simulink model "HEV_Model_PCT"  (R2014a)
settings: Solver=ode15s  StartTime=0.0  StopTime=195  RelTol=1e-5  AbsTol=1e-4
PreLoadFcn:
  | load UrbanCycle1
  | load UrbanCycle2
  | load UrbanCycle3
  | load UrbanCycle4
  | load UrbanCycle5
  | 
  | assignin('base','decimation',1)
  | Pbatt = 21e3;
  | Vbatt =100;
  | Ts = 6e-5;   % time step
  | 
  | Drive_Cycle_Num = 1;
PostLoadFcn:
  | warning off Simulink:SL_UsingDefaultMaxStepSize
  | warning off Simulink:blocks:MatchingGotoNotFound
  | warning off Simulink:blocks:MatchingFromNotFound
  | warning off Simulink:blocks:TDelayBufferTooSmall
  | warning off Simulink:SL_SaveWithParameterizedLinks_Warning
  | warning off Simulink:SL_TDelayBufferTooSmall
  | warning off ne_sli:nesl_compile:SolverNotRecommended
  | warning off Simulink:SL_OutputNotConnected
  | warning off Simulink:SL_SetParamLinkChangeWarn
  | warning off Simulink:SL_SaveWithDisabledLinks_Warning
  | warning('off','Simulink:SL_UINotUpdatedDuringRapidAccelSim');
  | warning off Simulink:Engine:OutputNotConnected
  | warning off Simulink:Engine:UINotUpdatedDuringRapidAccelSim
  | warning off Simulink:Engine:SaveWithParameterizedLinks_Warning
  | warning off Simulink:Engine:SolverMaskedZC
  | set_param(bdroot,'MaskedZcDiagnostic','none');
  | warning off Simulink:Engine:SolverInconsistentInitialConditionsWarnForDAE
  | set_param(bdroot,'IgnoredZcDiagnostic','none');
  | warning off Simulink:Engine:SolverIgnoredZCBracketing
  | set_param(bdroot,'MaxConsecutiveZCsMsg','none');
  | warning off Simulink:Engine:SolverConsecutiveZCNum
  | warning off Simulink:Engine:SolverMinStepSizeWarnForDAE
  | 
  | %Setup_HEV_Model_Configurations
InitFcn:
  | %Configure_HEV_Simulation
model workspace (MAT data in the model file):
  guiH = 18054.0001221
undefined symbols (not defined in the file or in its folder): drive_block, drive_enginemodel, HEV_Param, HEV_Vehicle_Dynamics_Lib, sigbuilder_block, Simple, speed, torque
undefined symbols (not defined in the file): HEV_Vehicle_Mass
libraries: fl_lib x34, nesl_utility x16, sdl_lib x2, simulink x1, HEV_Electrical_Lib x1, TunableMech_lib x1, powerlib x1
(part 1 of 2)
Description:
  | Copyright 2008 The MathWorks(TM), Inc.
settings Model: ExtModeAutoUpdateStatusClock=off  TunableVars=Drive_Cycle_Num,HEV_Vehicle_Mass  TunableVarsStorageClass=Auto,Auto  TunableVarsTypeQualifier=,  BufferReuse=off  Creator=tegel  LastModifiedBy=smiller
settings SolverCC: ZcThreshold=0  ZeroCrossAlgorithm=Adaptive
settings DataIOCC: SignalLoggingSaveFormat=ModelDataLogs  DSMLogging=off
settings OptimizationCC: InlineParams=on  OptimizeBlockIOStorage=off  BufferReuse=off  GlobalBufferReuse=off  ExpressionFolding=off  ExpressionDepthLimit=2147483647  LocalBlockOutputs=off  InitFltsAndDblsToZero=on  EfficientMapNaN2IntZero=off
settings DebuggingCC: AlgebraicLoopMsg=error  UnderspecifiedInitializationDetection=Classic  SignalResolutionControl=TryResolveAllWithWarning  MaxConsecutiveZCsMsg=none  MaskedZcDiagnostic=none  IgnoredZcDiagnostic=none  MultiTaskDSMMsg=warning  MultiTaskCondExecSysMsg=none  SigSpecEnsureSampleTimeMsg=none  FcnCallInpInsideContextMsg=UseLocalSettings  UnknownTsInhSupMsg=none  StateNameClashWarn=warning
settings HardwareCC: TargetLongLongMode=on  TargetEndianess=LittleEndian  TargetHWDeviceType=MATLAB Host  ProdEqTarget=off
settings SFSimCC: SimParseCustomCode=off
settings GRTTargetCC: CombineOutputUpdateFcns=off  GRTInterface=on

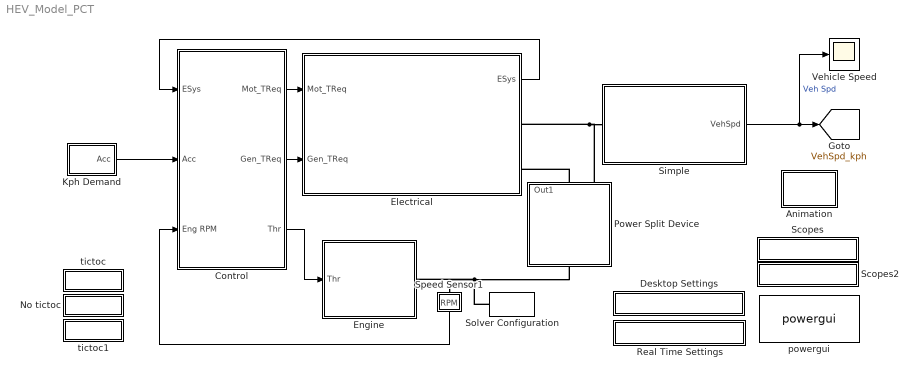
== system HEV_Model_PCT ==
  Animation : Subsystem  BlockChoice=Off
      mask init:
      | Configure_HEV_Animation
      settings: AttributesFormatString=%<BlockChoice>  TemplateBlock=Animation_Lib/Animation  MemberBlocks=Off,On
  Control : Subsystem
      mask Display:
      | image(imread('HEV_Control_IMAGE.jpg'));
      | port_label('input',1,'ESys');
      | port_label('input',2,'Acc');
      | port_label('input',3,'Eng RPM');
      | port_label('output',1,'Mot_TReq');
      | port_label('output',2,'Gen_TReq');
      | port_label('output',3,'Thr');
  Desktop Settings : Subsystem
      settings: OpenFcn=|
      | set_param(bdroot,'Solver','ODE15s');
      | 
      | %set_param([bdroot '/Electrical'],'MaskInitialization','Configure_HEV_Simulation');
      | 
      | %set_param([bdroot '/Animation'],'MaskInitialization','Configure_HEV_Simulation');
      | 
      | HEV_Param.Control.Mode_Logic_TS = 0.1;
      | 
      | tvar_solverBlock = find_system(bdroot,'FollowLinks','on','LookUnderMasks','on', 'SubClassName', 'solver');
      | 
      | for i=1:size(tvar_solverBlock,1)
      | 
      | set_param(char(tvar_solverBlock(i)), 'UseLocalSolver','off','DoFixedCost','off');
      | end
      | 
      | clear tvar_solverBlock
      mask Display: disp('Desktop Settings')
  Electrical : Subsystem  BlockChoice=System Level
      link override Detailed/Battery: BlockChoice=Predefined
      link override System Level/Battery: BlockChoice=Generic
      link override System Level/Battery/Predefined/Intf: T=100000
      link override System Level/Battery/Predefined/Preset Battery: SOC=HEV_Param.Battery_Det.Initial_SOC  MaxQ=8.1  FullV=232.7974  Dis_rate=3.5217  R=0.24691  Normal_OP=7.3252  expZone="[216.0772     0.3979565]"  Dis_Char=off  NomV=HEV_Param.Battery_Det.Nominal_Voltage  BatType=Nickel-Metal-Hydride
      mask init:
      | %disp('Elec Mask Init');
      | Configure_HEV_Simulation
      settings: AttributesFormatString=%<BlockChoice>  TemplateBlock=HEV_Electrical_Lib/Electrical  MemberBlocks=Detailed,Mean Value,System Level
  Engine : Subsystem
      mask Display:
      | image(imread('HEV_Engine_IMAGE.jpg'));
      | port_label('input',1,'Thr');
      | port_label('RConn',1,'Sh');
  Kph Demand : Subsystem
      mask Display:
      | plotstr=['UrbanCycle' evalin('base','num2str(Drive_Cycle_Num)')];
      | plot(evalin('base',[plotstr '.time']),evalin('base',[plotstr '.SpdKph']));
      | text(evalin('base',['0.7*max(' plotstr '.time)']),evalin('base',['0.25*max(' plotstr '.SpdKph)']),evalin('base','num2str(Drive_Cycle_Num)'));
  No tictoc : Subsystem
      settings: OpenFcn=|
      | set_param(bdroot,'StartFcn','');
      | set_param(bdroot,'StopFcn','');
      mask Display: disp('No tictoc')
  "Power Split Device " : Subsystem
      mask Display:
      | image(imread('HEV_Planetary_Gear_IMAGE.jpg'));
      | color('black');
      | port_label('Lconn',1,'C');
      | port_label('Rconn',1,'S');
      | port_label('Rconn',2,'R');
  Real Time Settings : Subsystem
      settings: OpenFcn=|
      | tvar_Nonlinear_Iterations = '3';
      | tvar_StepSize = '0.005';                                                                                                                                                                               Select_HEV_Model_Systems('Sys BC VS',HEV_Configs);
      | 
      | %tvar_LocalSolver = 'NE_TRAPEZOIDAL_ADVANCER';
      | tvar_LocalSolver = 'NE_BACKWARD_EULER_ADVANCER';
      | 
      | set_param([bdroot '/Electrical'],'MaskInitialization','%Configure_HEV_Simulation');                                                                                                                set_param([bdroot '/Animation'],'MaskInitialization','%Configure_HEV_Simulation');
      | 
      | HEV_Param.Control.Mode_Logic_TS = str2num(tvar_StepSize);
      | 
      | set_param(bdroot,'Solver','ode1','FixedStep','auto');
      | tvar_solverBlock = find_system(bdroot,'FollowLinks','on','LookUnderMasks','on', 'SubClassName', 'solver');
      | for i=1:size(tvar_solverBlock,1)
      | 
      | 
      |     set_param(char(tvar_solverBlock(i)), 'UseLocalSolver','on','DoFixedCost','on','MaxNonlinIter',tvar_Nonlinear_Iterations,'LocalSolverChoice',tvar_LocalSolver,'LocalSolverSampleTime',tvar_StepSize);
      | end
      | clear tvar_Nonlinear_Iterations tvar_StepSize tvar_LocalSolver tvar_solverBlock
      mask Display: disp('Real Time Settings')
  Scopes : Subsystem  mask(Data Acquisition){}
      mask Display: disp('Scopes');
  Scopes2 : Subsystem  mask(Data Acquisition){}
      mask Display: disp('Fuel Economy');
  Simple : Subsystem  AncestorBlock=HEV_Vehicle_Dynamics_Lib/Simple  mask(Rigid vehicle model){mass=HEV_Vehicle_Mass, area=HEV_Param.Vehicle.Frontal_Area, Cd=HEV_Param.Vehicle.Aero_Drag_Coeff, radius=HEV_Param.Vehicle.Tire_Radius, wheel_inertia=HEV_Param.Vehicle.Wheel_Inertia, gear_ratio=HEV_Param.Vehicle.Engine_Vehicle_Gear_Ratio}
      mask prompts: mass "Vehicle mass (Kg)"; area "Vehicle Area (m^2)"; Cd "Aerodynamic drag coefficient (unitless)"; radius "Tire radius (m)"; wheel_inertia "Total wheel inertia (kg*m^2)"; gear_ratio "Engine to vehicle gear ratio"
      mask help:
      | Model vehicle effective inertia and drag force as seen by the engine. It
      | is assumed that the vehicle is moving on flat terrain. No bearing friction
      | or gear losses are included.
      mask init:
      | gravity = 9.81;
      mask Display:
      | image(imread('HEV_Vehicle_Dynamics_Simple_IMAGE.jpg'));
      | port_label('LConn',1,'Sh');
      | port_label('output',1,'Spd');
  Solver Configuration : nesl_utility/Solver Configuration  PhysicalDomain=network_engine_domain  SubClassName=solver  LeftPortType=input  RightPortType=generic  Accelerate=off  Tones=[]  Harmonics=[]  SimulateNoise=off  Profile=off  UseLocalSampling=off  EnableSwitchedLinearOptims=on  FrequencyDomain=off  UseCCode=off  RelTol=0.001  AbsTol=1e-06  MinStep=1e-09  ToWorkspace=off  DoDC=off  ResidualTolerance=1e-8  UseLocalSolver=off  LocalSolverChoice=NE_BACKWARD_EULER_ADVANCER  LocalSolverSampleTime=0.005  DoFixedCost=off  MaxNonlinIter=3  MaxModeIter=2  LinearAlgebra=Sparse  DelaysMemoryBudget=1024  AutomaticFiltering=on  FilteringTimeConstant=0.001
  Speed Sensor1 : Subsystem
      mask Display: disp('S')
  Vehicle Speed : Scope
      settings: YMin=-20  YMax=120  Decimation=decimation
  powergui : powerlib/powergui  SimulationMode=Continuous  SolverType=Tustin  SampleTime=Ts  frequency=60  SPID=on  DisableSnubberDevices=off  DisableRonSwitches=off  DisableVfSwitches=off  SwTol=0  Interpol=off  DisplayEquations=off  Ts=0  methode=off  frequencyindice=0  Pbase=100e6  ErrMax=1e-4  Iterations=50  UnitsV=kV  UnitsW=MW  FunctionMessages=off  echomessages=off  HookPort=off  EnableUseOfTLC=off  x0status=blocks  RestoreLinks=warning  ResistiveCurrentMeasurement=off  Frange=[0:2:500]  Ylog=off  Xlog=on  ShowGrid=off  save=off  variable=ZData  structure=0  ZoomFFT=on  StartTime=0.0  cycles=1  DisplayStyle=1  fundamental=60  FreqAxis=off  MaxFrequency=1000  frequencyindicesteady=1  RmsSteady=1  display=off
  tictoc : Subsystem
      settings: OpenFcn=|
      | set_param(bdroot,'StartFcn','tic;');
      | set_param(bdroot,'StopFcn','Elapsed_Sim_Time = toc; disp([''Elapsed time is '' num2str(Elapsed_Sim_Time)])');
      mask Display: disp('tictoc')
  tictoc1 : Subsystem
      settings: OpenFcn=open('HEV_Model_Demo_Script.html')
      mask Display: disp('Script')
  tag scope: VehSpd_kph=global
  wires:
  Simple/1(VehSpd) -> [VehSpd_kph], Vehicle Speed/1  "Veh Spd"
  Speed Sensor1/1(RPM) -> Control/3(Eng RPM)
  Control/1(Mot_TReq) -> Electrical/1(Mot_TReq)
  Control/2(Gen_TReq) -> Electrical/2(Gen_TReq)
  Control/3(Thr) -> Engine/1(Thr)
  Kph Demand/1(Acc) -> Control/2(Acc)
  Electrical/1(ESys) -> Control/1("ESys ")
  connections:
  "Power Split Device "/RConn1 -- Electrical/RConn2
  Simple/LConn1 -- "Power Split Device "/RConn2 -- Electrical/RConn1
  Engine/RConn1 -- Speed Sensor1/LConn1 -- "Power Split Device "/LConn1 -- Solver Configuration/RConn1

== system HEV_Model_PCT/Animation ==
  Off : Subsystem

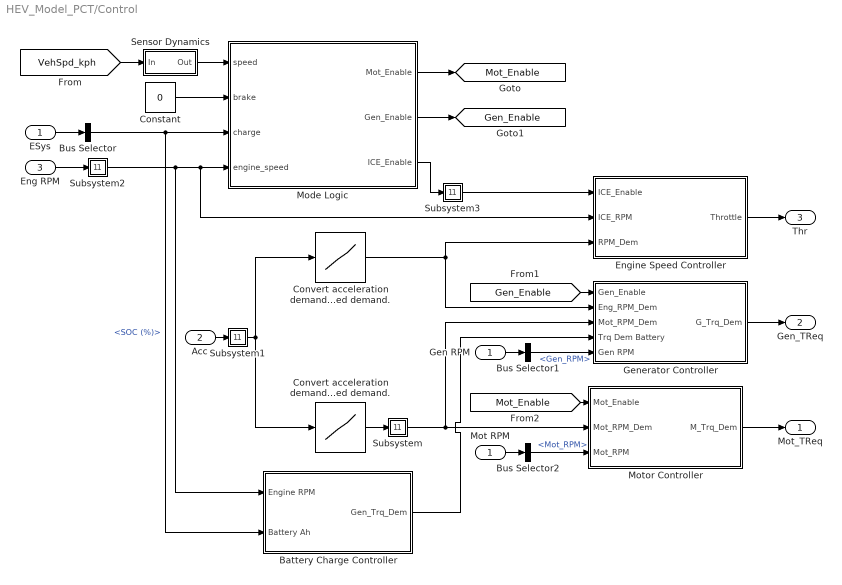
== system HEV_Model_PCT/Control ==
  "ESys " : Inport
  Acc : Inport  Port=2
  Eng RPM : Inport  Port=3
  Battery Charge Controller : Subsystem
  Bus Selector : BusSelector  OutputSignals=Batt.SOC (%)
  Bus Selector1 : BusSelector  OutputSignals=Gen_RPM
  Bus Selector2 : BusSelector  OutputSignals=Mot_RPM
  Constant : Constant  Value=0
  Convert acceleration demand to engine speed demand. : Lookup  InputValues=[0 0.1 1]  Table=[0 800 4000]
  Convert acceleration demand to motor speed demand. : Lookup  InputValues=[0 1]  Table=[0 2500]
  Engine Speed Controller : Subsystem
  Gen RPM : InportShadow
  Generator Controller : Subsystem
  Mode Logic : Stateflow chart  TreatAsAtomicUnit=on
  Mot RPM : InportShadow
  Motor Controller : Subsystem
  Sensor Dynamics : Subsystem  mask(First-order lag supporting vector signals){b=HEV_Param.ICE.sensor_time_constant, x_initial=0}
      mask prompts: b "Filter time constant"; x_initial "Initial output"
      mask help: Models a lag of the form 1/(b*s+1) where s is the Laplace operator.
  Subsystem : Subsystem
      mask Display: disp('S')
  Subsystem1 : Subsystem
      mask Display: disp('S')
  Subsystem2 : Subsystem
      mask Display: disp('S')
  Subsystem3 : Subsystem
      mask Display: disp('S')
  Mot_TReq : Outport
  Gen_TReq : Outport  Port=2
  Thr : Outport  Port=3
  tag scope: Gen_Enable=global, Mot_Enable=global
  wires:
  Acc/1 -> Subsystem1/1(In1)
  Eng RPM/1 -> Subsystem2/1(In1)
  Engine Speed Controller/1(Throttle) -> Thr/1
  Convert acceleration demand to motor speed demand./1 -> Subsystem/1(In1)
  Convert acceleration demand to engine speed demand./1 -> Engine Speed Controller/3(RPM_Dem), Generator Controller/2(Eng_RPM_Dem)
  Bus Selector2/1 -> Motor Controller/3(Mot_RPM)  "<Mot_RPM>"
  Motor Controller/1(M_Trq_Dem) -> Mot_TReq/1
  Generator Controller/1(G_Trq_Dem) -> Gen_TReq/1
  "ESys "/1 -> Bus Selector/1
  Subsystem2/1(Eng_RPM_Meas) -> Battery Charge Controller/1(Engine RPM), Mode Logic/4(engine_speed), Engine Speed Controller/2(ICE_RPM)
  Bus Selector/1 -> Battery Charge Controller/2(Battery Ah), Mode Logic/3(charge)  "<SOC (%)>"
  Constant/1 -> Mode Logic/2(brake)
  Mode Logic/3(ICE_Enable) -> Subsystem3/1(In1)
  Subsystem3/1(Gen_RPM_Dem) -> Engine Speed Controller/1(ICE_Enable)
  Mode Logic/2(Gen_Enable) -> [Gen_Enable]
  Mode Logic/1(Mot_Enable) -> [Mot_Enable]
  Sensor Dynamics/1(Out) -> Mode Logic/1(speed)
  Bus Selector1/1 -> Generator Controller/5(Gen RPM)  "<Gen_RPM>"
  Subsystem/1(Motor_RPM_Dem) -> Motor Controller/2(Mot_RPM_Dem), Generator Controller/3(Mot_RPM_Dem)
  [Gen_Enable] -> Generator Controller/1(Gen_Enable)
  [Mot_Enable] -> Motor Controller/1(Mot_Enable)
  Battery Charge Controller/1(Gen_Trq_Dem) -> Generator Controller/4(Trq Dem Battery)
  Gen RPM/1 -> Bus Selector1/1
  Mot RPM/1 -> Bus Selector2/1
  Subsystem1/1(Accel) -> Convert acceleration demand to motor speed demand./1, Convert acceleration demand to engine speed demand./1
  [VehSpd_kph] -> Sensor Dynamics/1(In)

== system HEV_Model_PCT/Desktop Settings ==

== system HEV_Model_PCT/Electrical ==
  Mot_TReq : Inport
  Gen_TReq : Inport  Port=2
  System Level : HEV_Electrical_Lib/System Level  SystemSampleTime=-1
  Mot_Sh : PMIOPort  Port=1  Side=Right
  Gen_Sh : PMIOPort  Port=2  Side=Right
  ESys : Outport
  wires:
  Mot_TReq/1 -> System Level/1
  Gen_TReq/1 -> System Level/2
  System Level/1 -> ESys/1
  connections:
  System Level/RConn1 -- Mot_Sh/RConn1
  System Level/RConn2 -- Gen_Sh/RConn1

== system HEV_Model_PCT/Engine ==
  Thr : Inport
  Generic Engine : sdl_lib/Engines/Generic Engine  model_parameterization=1  engine_type=1  P_max=HEV_Param.ICE.Max_Power W  w_P_max=HEV_Param.ICE.Speed_At_Max_Power rpm  w_max=HEV_Param.ICE.Max_Speed rpm  w_min=500 rpm  w_tab=[ 500 1000 2e+3 3e+3 4e+3 5e+3 6e+3 7e+3 ] rpm  trq_tab=[ 380 380 380 380 350 280 200 80 ] N*m  pwr_tab=[ 2e+4 4e+4 7.8e+4 1.2e+5 1.45e+5 1.48e+5 1.25e+5 6e+4 ] W  interp_method=1  model_inertia=0  inertia=1 kg*m^2  initial_velocity=800 rpm  model_time_constant=0  time_constant=0.2 s  T0=0  w_thr=100 rpm  idle_speed=0  idle_speed_reference=1000 rpm  tau_controller=1 s  idle_w_thr=1 rpm  fc_model=1  fc_per_rev=25 mg/rev  displaced_volume=400 cm^3  rev_per_cycle=2  fc_w_tab=[ 1000 2e+3 3e+3 4e+3 5e+3 6e+3 ] rpm  fc_trq_tab=[ 0 80 160 200 240 320 360 400 ] N*m  fc_tab=[ 0.5 0.9 1.4 1.6 1.9 2.7 3.4 4.4; 1 1.7 2.7 3.1 3.6 5 6 7.4; 1.4 2.7 4 4.8 5.6 7.5 8.5 10.5; 2 3.6 5.8 6.7 8 10.4 11.7 13.3; 2.5 4.8 7.9 9.4 10.8 14 16.2 18.6; 3.1 6 10.3 11.9 13.8 18.4 22 26.5 ] g/s  bmep_tab=[ 0 250 500 625 750 1000 1.15e+3 1.25e+3 ] kPa  bsfc_tab=[ 410 380 300 280 270 290 320 380; 410 370 290 270 260 270 285 320; 415 380 290 275 265 270 270 300; 420 390 310 290 285 280 280 285; 430 410 340 320 310 300 310 320; 450 430 370 340 330 330 350 380 ] g/hr/kW  fc_interp_method=1
  Inertia1 : fl_lib/Mechanical/Rotational Elements/Inertia  inertia=HEV_Param.ICE.Shaft_Inertia kg*m^2  w_specify=on  w_priority=High  w=0 rad/s  t_specify=off  t_priority=High  t=0 N*m
  Mechanical Rotational Reference : fl_lib/Mechanical/Rotational Elements/Mechanical Rotational Reference
  Mechanical Rotational Reference1 : fl_lib/Mechanical/Rotational Elements/Mechanical Rotational Reference
  Rotational Damper : fl_lib/Mechanical/Rotational Elements/Rotational Damper  D=HEV_Param.ICE.Friction N*m/(rad/s)  w_specify=off  w_priority=High  w=0 rad/s  t_specify=off  t_priority=High  t=0 N*m
  Sensor : Subsystem
      mask Display: disp('S');
  Simulink-PS Converter : nesl_utility/Simulink-PS Converter  PhysicalDomain=network_engine_domain  SubClassName=ps_input  LeftPortType=input  RightPortType=output  PseudoPeriodic=off  Frequencies=[]  NoiseDistribution=none  NoiseParameters=[]  Unit=1  AffineConversion=off  InputFiltering=off  SimscapeFilterOrder=1  InputFilterTimeConstant=.001  UdotUserProvided=0
  Sh : PMIOPort  Port=1  Side=Right
  wires:
  Thr/1 -> Simulink-PS Converter/1  "Throttle"
  connections:
  Sensor/RConn1 -- Sh/RConn1
  Mechanical Rotational Reference1/LConn1 -- Rotational Damper/RConn1
  Simulink-PS Converter/RConn1 -- Generic Engine/LConn1
  Mechanical Rotational Reference/LConn1 -- Generic Engine/LConn2
  Sensor/LConn1 -- Generic Engine/RConn3 -- Inertia1/LConn1 -- Rotational Damper/LConn1

== system HEV_Model_PCT/Kph Demand ==
  "10-15 mode " : Subsystem  Tag=STV Subsys  LoadFcn=sigbuilder_block('load');  StartFcn=sigbuilder_block('start');  StopFcn=sigbuilder_block('stop');  ClipboardFcn=sigbuilder_block('clipboard');  mask(Sigbuilder block){}
      mask help: Sigbuilder GUI
      mask init:
      | if ~strcmp(get_param(bdroot(gcbh),'SimulationStatus'),'stopped') tuvar = sigbuilder_block('maskInit'); end
      settings: CopyFcn=sigbuilder_block('copy');  DeleteFcn=sigbuilder_block('delete');  ModelCloseFcn=sigbuilder_block('modelClose');  PreSaveFcn=sigbuilder_block('preSave');  PauseFcn=sigbuilder_block('pause')  ContinueFcn=sigbuilder_block('continue')  NameChangeFcn=sigbuilder_block('namechange');  OpenFcn=sigbuilder_block('open',[561.75 178.5 550.5 399 ]);  CloseFcn=sigbuilder_block('close');
      mask Display: plot(0,0,100,100,[10,10,40,40,10],[80,20,20,80,80],[40,10],[50,50], [40,27,10],[65,72,56],[40,25,25,10],[28,28,43,43]);
  FTP75 : FromWorkspace  VariableName=[UrbanCycle4.time UrbanCycle4.SpdKph]  SampleTime=0
  Multiport Switch : MultiPortSwitch  Inputs=5
  Select Cycle : Constant  Value=Drive_Cycle_Num
  Urban Cycle 1 : FromWorkspace  VariableName=[UrbanCycle1.time UrbanCycle1.SpdKph]  SampleTime=0
  Urban Cycle 2 : FromWorkspace  VariableName=[UrbanCycle2.time UrbanCycle2.SpdKph]  SampleTime=0
  Urban Cycle 3 : FromWorkspace  VariableName=[UrbanCycle3.time UrbanCycle3.SpdKph]  SampleTime=0
  Vehicle Speed Controller : Subsystem
  Acc : Outport
  wires:
  Urban Cycle 3/1 -> Multiport Switch/4
  Select Cycle/1 -> Multiport Switch/1
  Urban Cycle 2/1 -> Multiport Switch/3
  Urban Cycle 1/1 -> Multiport Switch/2
  Vehicle Speed Controller/1(Acc) -> Acc/1
  Multiport Switch/1 -> Vehicle Speed Controller/1(Ref Spd)
  [VehSpd_kph] -> Vehicle Speed Controller/2(Veh Spd)
  FTP75/1 -> Multiport Switch/5
  "10-15 mode "/1(Target speed) -> Multiport Switch/6

== system HEV_Model_PCT/No tictoc ==

== system HEV_Model_PCT/Power Split Device  ==
  note: For port placement
  Constant : Constant
  Planetary Gear : sdl_lib/Gears/Planetary Gear  rs_ratio=HEV_Param.Power_Split.Ratio_Ring2Sun  friction_model=2  efficiency=[ 0.96 0.98 ]  mu_visc=[ 0.02 0 ] N*m/(rad/s)  w_thr=[ 0.01 0.01] rad/s
  Sensor1 : Subsystem
      mask Display: disp('S')
  Sensor2 : Subsystem
      mask Display: disp('S')
  Sensor3 : Subsystem
      mask Display: disp('S')
  S : PMIOPort  Port=1  Side=Right
  R : PMIOPort  Port=2  Side=Right
  C : PMIOPort  Port=3  Side=Left
  Out1 : Outport
  wires:
  Constant/1 -> Out1/1
  connections:
  S/RConn1 -- Sensor3/RConn1
  Planetary Gear/RConn1 -- Sensor2/LConn1
  Planetary Gear/RConn2 -- Sensor3/LConn1
  R/RConn1 -- Sensor2/RConn1
  Sensor1/LConn1 -- C/RConn1
  Sensor1/RConn1 -- Planetary Gear/LConn1

== system HEV_Model_PCT/Real Time Settings ==

== system HEV_Model_PCT/Scopes ==
  Batt Cell Temp : Scope
      settings: YMin=20  YMax=60  SaveName=DCDC_Temp1  MaxDataPoints=100  Decimation=decimation
  Batt DCDC Scopes : Subsystem
  Car Scopes : Subsystem
  DC DC Temp : Scope
      settings: YMin=20  YMax=60  SaveName=DCDC_Temp  MaxDataPoints=100  Decimation=decimation*100
  Demux1 : Demux  Outputs=2
  Drivetrain Scopes : Subsystem
  Electricals Scopes : Subsystem
  ICE Scopes : Subsystem
  Mode Logic : Subsystem
  Motor Generator Scopes : Subsystem
  Speeds (RPM) : Scope  NumInputPorts=2
      settings: YMin=-500~-1000  YMax=1500~5000  SaveName=ScopeData9  MaxDataPoints=100  Decimation=decimation
  Voltages : Scope  NumInputPorts=2
      settings: YMin=490~160  YMax=520~260  MaxDataPoints=100  Decimation=decimation
  wires:
  Electricals Scopes/1(V) -> Demux1/1
  Demux1/1 -> Voltages/1  "DC Bus"
  Demux1/2 -> Voltages/2  "Battery"
  Motor Generator Scopes/1(M) -> Speeds (RPM)/1  "Motor"
  Motor Generator Scopes/2(G) -> Speeds (RPM)/2  "Generator"
  Batt DCDC Scopes/1(DCDC Temp) -> DC DC Temp/1
  Batt DCDC Scopes/2(Batt Cell Temp) -> Batt Cell Temp/1

== system HEV_Model_PCT/Scopes2 ==
  note: Fuel Economy
  (L/100 km) : Display
      settings: Decimation=decimation
  (MPG) : Display
      settings: Decimation=decimation
  (km/L) : Display
      settings: Decimation=decimation
  Calculate Fuel Economy : Subsystem
  Fuel Consumption Table : Lookup2D  RowIndex=HEV_Param.ICE.FC.Speed_Vector  ColumnIndex=HEV_Param.ICE.FC.Torque_Vector  Table=HEV_Param.ICE.FC.Consumption_Table
  Total Fuel Used (L) : Display
      settings: Decimation=decimation
  wires:
  Calculate Fuel Economy/1(Liter/100Km) -> (L/100 km)/1
  Calculate Fuel Economy/3(MPG) -> (MPG)/1
  [VehSpd_kph] -> Calculate Fuel Economy/1(Kph)
  Calculate Fuel Economy/4(Fuel Used (L)) -> Total Fuel Used (L)/1
  Calculate Fuel Economy/2(Km/Liter) -> (km/L)/1
  Fuel Consumption Table/1 -> Calculate Fuel Economy/2(Fuel Flow g/s)
  [EngSpd_RPM] -> Fuel Consumption Table/1
  [Carrier_Trq_Nm] -> Fuel Consumption Table/2

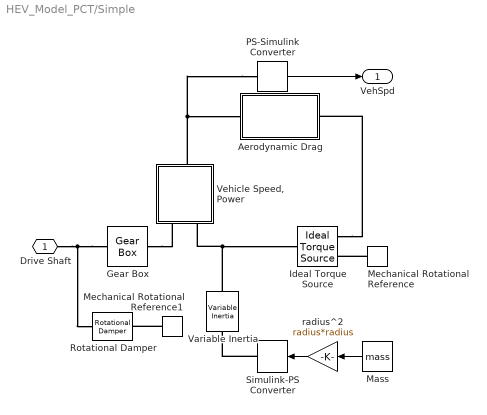
== system HEV_Model_PCT/Simple ==
  Aerodynamic Drag : Subsystem
  Gear Box : fl_lib/Mechanical/Mechanisms/Gear Box  ratio=gear_ratio  t_in_specify=off  t_in_priority=High  t_in=0 N*m  t_out_specify=off  t_out_priority=High  t_out=0 N*m
  Ideal Torque Source : fl_lib/Mechanical/Mechanical Sources/Ideal Torque Source
  Mass : Constant  Value=mass
  Mechanical Rotational Reference : fl_lib/Mechanical/Rotational Elements/Mechanical Rotational Reference
  Mechanical Rotational Reference1 : fl_lib/Mechanical/Rotational Elements/Mechanical Rotational Reference
  PS-Simulink Converter : nesl_utility/PS-Simulink Converter  PhysicalDomain=network_engine_domain  SubClassName=ps_output  LeftPortType=input  RightPortType=output  PseudoPeriodic=off  Frequencies=[]  Unit=1  AffineConversion=off
  Rotational Damper : fl_lib/Mechanical/Rotational Elements/Rotational Damper  D=HEV_Param.Vehicle.Trans.Friction N*m/(rad/s)  w_specify=off  w_priority=High  w=0 rad/s  t_specify=off  t_priority=High  t=0 N*m
  Simulink-PS Converter : nesl_utility/Simulink-PS Converter  PhysicalDomain=network_engine_domain  SubClassName=ps_input  LeftPortType=input  RightPortType=output  PseudoPeriodic=off  Frequencies=[]  NoiseDistribution=none  NoiseParameters=[]  Unit=kg*m*m  AffineConversion=off  InputFiltering=off  SimscapeFilterOrder=1  InputFilterTimeConstant=.001  UdotUserProvided=0
  Variable Inertia : TunableMech_lib/Variable Inertia  initial_velocity=0 rad/s  t_specify=off  t_priority=High  t=0 N*m
  "Vehicle Speed, Power" : Subsystem
  radius^2 : Gain  Gain=radius*radius
  Drive Shaft : PMIOPort  Port=1  Side=Left
  VehSpd : Outport
  wires:
  PS-Simulink Converter/1 -> VehSpd/1
  Mass/1 -> radius^2/1
  radius^2/1 -> Simulink-PS Converter/1
  connections:
  Gear Box/RConn1 -- "Vehicle Speed, Power"/LConn1
  Mechanical Rotational Reference1/LConn1 -- Rotational Damper/RConn1
  Variable Inertia/LConn1 -- "Vehicle Speed, Power"/LConn2 -- Ideal Torque Source/LConn1
  Mechanical Rotational Reference/LConn1 -- Ideal Torque Source/RConn2
  Ideal Torque Source/RConn1 -- Aerodynamic Drag/RConn1
  PS-Simulink Converter/LConn1 -- Aerodynamic Drag/LConn1 -- "Vehicle Speed, Power"/RConn1
  Gear Box/LConn1 -- Drive Shaft/RConn1 -- Rotational Damper/LConn1
  Simulink-PS Converter/RConn1 -- Variable Inertia/RConn1

== system HEV_Model_PCT/Speed Sensor1 ==
  Ideal Rotational Motion Sensor : fl_lib/Mechanical/Mechanical Sensors/Ideal Rotational Motion Sensor  offset=0 rad
  Mechanical Rotational Reference : fl_lib/Mechanical/Rotational Elements/Mechanical Rotational Reference
  PS-Simulink Converter1 : nesl_utility/PS-Simulink Converter  PhysicalDomain=network_engine_domain  SubClassName=ps_output  LeftPortType=input  RightPortType=output  PseudoPeriodic=off  Frequencies=[]  Unit=rpm  AffineConversion=off
  Sensor Dynamics : Subsystem  mask(First-order lag supporting vector signals){b=HEV_Param.ICE.sensor_time_constant, x_initial=0}
      mask prompts: b "Filter time constant"; x_initial "Initial output"
      mask help: Models a lag of the form 1/(b*s+1) where s is the Laplace operator.
  Shaft : PMIOPort  Port=1  Side=Left
  RPM : Outport
  wires:
  PS-Simulink Converter1/1 -> Sensor Dynamics/1(In)
  Sensor Dynamics/1(Out) -> RPM/1
  connections:
  PS-Simulink Converter1/LConn1 -- Ideal Rotational Motion Sensor/RConn2
  Mechanical Rotational Reference/LConn1 -- Ideal Rotational Motion Sensor/RConn1
  Ideal Rotational Motion Sensor/LConn1 -- Shaft/RConn1

== system HEV_Model_PCT/tictoc ==

== system HEV_Model_PCT/tictoc1 ==

== system HEV_Model_PCT/Animation/Off ==

== system HEV_Model_PCT/Control/Battery Charge Controller ==
  Engine RPM : Inport
  Battery Ah : Inport  Port=2
  Allow 20% of available torque to be used to charge the battery : Gain  Gain=-0.2
  Engine Model : Subsystem  DialogController=PMDialogs.PMDefaultMaskDlg  LoadFcn=drive_block('LoadFcn');  StartFcn=drive_enginemodel('Start');  mask(Gasoline Engine){power_max=43e3, speed_at_power_max=4000, speed_max=6000}
      mask prompts: power_max "Maximum power [W]:"; speed_at_power_max "Speed at maximum power [rpm]:"; speed_max "Maximum speed [rpm]:"
      mask help:
      | Simple gasoline fuel engine model with speed governor.  The throttle input signal lies between zero and one and specifies the torque demanded from the engine as a fraction of the maximum possible torque.  This signal also indirectly controls the engine speed.  The engine model does not include air-fuel combustion dynamics.
      |
      | If the throttle signal rises above one or falls below zero, the engine limits the signal to one or zero, respectively. If the engine speed rises above the maximum speed, the engine torque drops to zero.
      mask init:
      | drive_preinitmask();[speed,power,torque,p] = ...
      | 	drive_enginemodel('MaskGasoline');
      settings: CopyFcn=drive_block('CopyFcn');  DeleteFcn=drive_block('DeleteFcn');  PreSaveFcn=drive_block('PreSaveFcn');  PostSaveFcn=drive_block('PostSaveFcn');  PreCopyFcn=drive_block('PreCopyFcn');  PreDeleteFcn=drive_block('PreDeleteFcn');
      mask Help: web(drive_help);
      mask Display:
      | image(imread('engine.bmp'),'center')
      | plot(speed, torque/max(torque))
      | plot(speed, power/max(power))
      | port_label('input', 1, 'RPM')
      | port_label('output', 1, 'Tmax')
  Engine-generator gear ratio : Gain  Gain=1/2
  "If the battery has more than 100% rated capacity, then no generation is required. Linearly ramp to using 20% of engine torque for charging between 50% capacity and 100% capacity." : Lookup  InputValues=[0 50 100 150]  Table=[-5 -5 0 0]
  Max : Constant  Value=5
  Nm2Volts : Gain  Gain=5/400
  Saturation Dynamic : simulink/Discontinuities/Saturation Dynamic  OutMin=[]  OutMax=[]  OutDataTypeStr=Inherit: Same as second input  OutDataType=sfix(16)  OutScaling=2^-10  DoSatur=off
  Volts2Nm : Gain  Gain=400/5
  Gen_Trq_Dem : Outport
  tag scope: gen_torque_dem=global
  wires:
  Battery Ah/1 -> "If the battery has more than 100% rated capacity, then no generation is required. Linearly ramp to using 20% of engine torque for charging between 50% capacity and 100% capacity."/1
  Engine RPM/1 -> Engine Model/1(RPM)
  Engine Model/1(Max Torque) -> Engine-generator gear ratio/1
  Allow 20% of available torque to be used to charge the battery/1 -> Nm2Volts/1  "Min Gen Trq (Nm)"
  Engine-generator gear ratio/1 -> Allow 20% of available torque to be used to charge the battery/1
  Nm2Volts/1 -> Saturation Dynamic/3  "Min torque controller demand (V)"
  Saturation Dynamic/1 -> Volts2Nm/1
  Max/1 -> Saturation Dynamic/1
  "If the battery has more than 100% rated capacity, then no generation is required. Linearly ramp to using 20% of engine torque for charging between 50% capacity and 100% capacity."/1 -> Saturation Dynamic/2
  Volts2Nm/1 -> Gen_Trq_Dem/1, [gen_torque_dem]

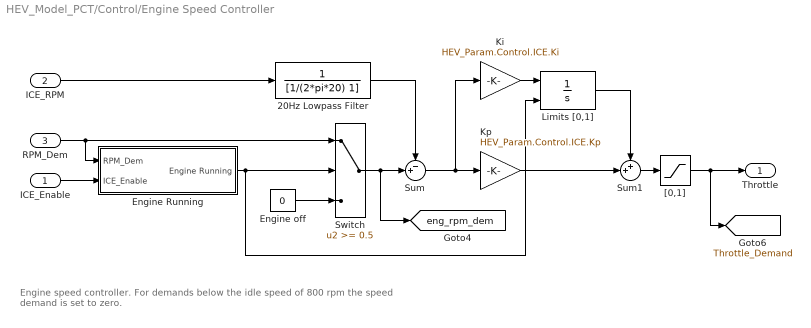
== system HEV_Model_PCT/Control/Engine Speed Controller ==
  note: Engine speed controller. For demands below the idle speed of
      | 800 rpm the speed demand is set to zero.
  ICE_Enable : Inport
  ICE_RPM : Inport  Port=2
  RPM_Dem : Inport  Port=3
  20Hz Lowpass Filter : TransferFcn  Denominator=[1/(2*pi*20) 1]
  Engine Running : Subsystem
  Engine off : Constant  Value=0
  Ki : Gain  Gain=HEV_Param.Control.ICE.Ki
  Kp : Gain  Gain=HEV_Param.Control.ICE.Kp
  Limits [0,1] : Integrator  ExternalReset=either  LimitOutput=on  UpperSaturationLimit=1  LowerSaturationLimit=0
  Sum : Sum  Inputs=-+|
  Sum1 : Sum  Inputs=++|
  Switch : Switch  Threshold=0.5
  "[0,1]" : Saturate  UpperLimit=1  LowerLimit=0
  Throttle : Outport
  tag scope: Throttle_Demand=global, eng_rpm_dem=global
  wires:
  RPM_Dem/1 -> Switch/1, Engine Running/1(RPM_Dem)
  ICE_RPM/1 -> 20Hz Lowpass Filter/1
  Sum/1 -> Ki/1, Kp/1
  Ki/1 -> Limits [0,1]/1
  Kp/1 -> Sum1/2
  Limits [0,1]/1 -> Sum1/1
  20Hz Lowpass Filter/1 -> Sum/1
  Switch/1 -> Sum/2, [eng_rpm_dem]
  "[0,1]"/1 -> Throttle/1, [Throttle_Demand]
  Sum1/1 -> "[0,1]"/1
  Engine off/1 -> Switch/3
  ICE_Enable/1 -> Engine Running/2(ICE_Enable)
  Engine Running/1(Engine Running) -> Switch/2, Limits [0,1]/2

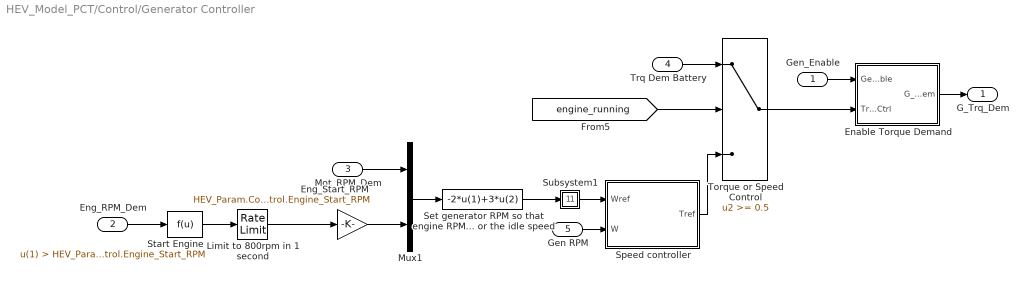
== system HEV_Model_PCT/Control/Generator Controller ==
  Gen_Enable : Inport
  Eng_RPM_Dem : Inport  Port=2
  Mot_RPM_Dem : Inport  Port=3
  Trq Dem Battery : Inport  Port=4
  Gen RPM : Inport  Port=5
  Enable Torque Demand : Subsystem
  Eng_Start_RPM : Gain  Gain=HEV_Param.Control.Engine_Start_RPM
  Limit to 800rpm in 1 second : RateLimiter  SampleTimeMode=inherited
  Mux1 : Mux  Inputs=2
  Set generator RPM so that engine RPM is controlled to zero or the idle speed : Fcn  Expr=-2*u(1)+3*u(2)
  Speed controller : Subsystem
  Start Engine : Fcn  Expr=u(1) > HEV_Param.Control.Engine_Start_RPM
  Subsystem1 : Subsystem
      mask Display: disp('S')
  Torque or Speed Control : Switch  Threshold=0.5
  G_Trq_Dem : Outport
  wires:
  Set generator RPM so that engine RPM is controlled to zero or the idle speed/1 -> Subsystem1/1(In1)
  Mux1/1 -> Set generator RPM so that engine RPM is controlled to zero or the idle speed/1
  Limit to 800rpm in 1 second/1 -> Eng_Start_RPM/1
  Eng_Start_RPM/1 -> Mux1/2
  Gen RPM/1 -> Speed controller/2(W)
  Speed controller/1(Tref) -> Torque or Speed Control/3
  Subsystem1/1(Gen_RPM_Dem) -> Speed controller/1(Wref)
  Start Engine/1 -> Limit to 800rpm in 1 second/1
  Mot_RPM_Dem/1 -> Mux1/1
  Eng_RPM_Dem/1 -> Start Engine/1
  Trq Dem Battery/1 -> Torque or Speed Control/1
  Gen_Enable/1 -> Enable Torque Demand/1(Gen_Enable)
  [engine_running] -> Torque or Speed Control/2
  Enable Torque Demand/1(G_Trq_Dem) -> G_Trq_Dem/1
  Torque or Speed Control/1 -> Enable Torque Demand/2(TrqDemCtrl)

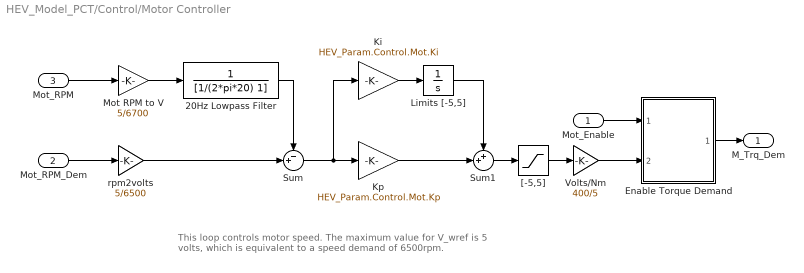
== system HEV_Model_PCT/Control/Motor Controller ==
  note: This loop controls motor speed. The maximum value
      | for V_wref is 5 volts, which is equivalent to a speed
      | demand of 6500rpm.
  Mot_Enable : Inport
  Mot_RPM_Dem : Inport  Port=2
  Mot_RPM : Inport  Port=3
  20Hz Lowpass Filter : TransferFcn  Denominator=[1/(2*pi*20) 1]
  Enable Torque Demand : Subsystem
  Ki : Gain  Gain=HEV_Param.Control.Mot.Ki
  Kp : Gain  Gain=HEV_Param.Control.Mot.Kp
  Limits [-5,5] : Integrator  LimitOutput=on  UpperSaturationLimit=5  LowerSaturationLimit=-5
  Mot RPM to V : Gain  Gain=5/6700
  Sum : Sum  Inputs=-+|
  Sum1 : Sum  Inputs=++|
  Volts/Nm : Gain  Gain=400/5
  "[-5,5]" : Saturate  UpperLimit=5  LowerLimit=-5
  rpm2volts : Gain  Gain=5/6500
  M_Trq_Dem : Outport
  wires:
  "[-5,5]"/1 -> Volts/Nm/1
  Mot_RPM/1 -> Mot RPM to V/1
  Sum1/1 -> "[-5,5]"/1
  Sum/1 -> Ki/1, Kp/1
  Ki/1 -> Limits [-5,5]/1
  Kp/1 -> Sum1/2
  Limits [-5,5]/1 -> Sum1/1
  20Hz Lowpass Filter/1 -> Sum/1
  rpm2volts/1 -> Sum/2
  Mot RPM to V/1 -> 20Hz Lowpass Filter/1
  Volts/Nm/1 -> Enable Torque Demand/2(TrqDemCtrl)
  Mot_RPM_Dem/1 -> rpm2volts/1
  Mot_Enable/1 -> Enable Torque Demand/1(Mot_Enable)
  Enable Torque Demand/1(TrqDem) -> M_Trq_Dem/1

== system HEV_Model_PCT/Control/Sensor Dynamics ==
  In : Inport
  Gain : Gain  Gain=1/b
  Integrator : Integrator  InitialCondition=x_initial
  Sum : Sum  Inputs=|+-  SaturateOnIntegerOverflow=on  InputSameDT=on  OutDataTypeStr=Inherit: Same as first input
  Out : Outport
  wires:
  Sum/1 -> Integrator/1
  In/1 -> Sum/1
  Integrator/1 -> Gain/1
  Gain/1 -> Sum/2, Out/1

== system HEV_Model_PCT/Control/Subsystem ==
  In1 : Inport
  Motor_RPM_Dem : Outport
  tag scope: motor_rpm_dem=global
  wires:
  In1/1 -> [motor_rpm_dem], Motor_RPM_Dem/1

== system HEV_Model_PCT/Control/Subsystem1 ==
  In1 : Inport
  Accel : Outport
  tag scope: Accelerator=global
  wires:
  In1/1 -> Accel/1, [Accelerator]

== system HEV_Model_PCT/Control/Subsystem2 ==
  In1 : Inport
  Eng_RPM_Meas : Outport
  tag scope: eng_rpm_meas=global
  wires:
  In1/1 -> Eng_RPM_Meas/1, [eng_rpm_meas]

== system HEV_Model_PCT/Control/Subsystem3 ==
  In1 : Inport
  Gen_RPM_Dem : Outport
  tag scope: ICE_Enable=global
  wires:
  In1/1 -> [ICE_Enable], Gen_RPM_Dem/1

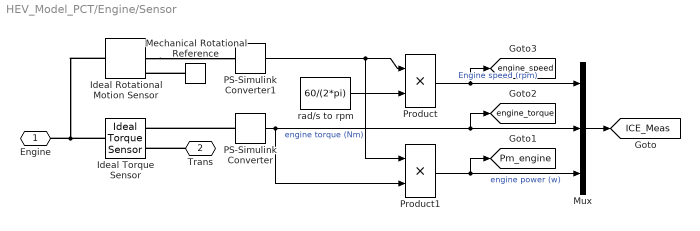
== system HEV_Model_PCT/Engine/Sensor ==
  Ideal Rotational Motion Sensor : fl_lib/Mechanical/Mechanical Sensors/Ideal Rotational Motion Sensor  offset=0 rad
  Ideal Torque Sensor : fl_lib/Mechanical/Mechanical Sensors/Ideal Torque Sensor
  Mechanical Rotational Reference : fl_lib/Mechanical/Rotational Elements/Mechanical Rotational Reference
  Mux : Mux  Inputs=3
  PS-Simulink Converter : nesl_utility/PS-Simulink Converter  PhysicalDomain=network_engine_domain  SubClassName=ps_output  LeftPortType=input  RightPortType=output  PseudoPeriodic=off  Frequencies=[]  Unit=N*m  AffineConversion=off
  PS-Simulink Converter1 : nesl_utility/PS-Simulink Converter  PhysicalDomain=network_engine_domain  SubClassName=ps_output  LeftPortType=input  RightPortType=output  PseudoPeriodic=off  Frequencies=[]  Unit=rad/s  AffineConversion=off
  Product : Product  RndMeth=Zero
  Product1 : Product  RndMeth=Zero
  rad/s to rpm : Constant  Value=60/(2*pi)
  Engine : PMIOPort  Port=1  Side=Left
  Trans : PMIOPort  Port=2  Side=Right
  tag scope: ICE_Meas=global, Pm_engine=global, engine_speed=global, engine_torque=global
  wires:
  PS-Simulink Converter/1 -> Product1/2, Mux/2, [engine_torque]  "engine torque (Nm)"
  Product1/1 -> Mux/3, [Pm_engine]  "engine power (w)"
  Product/1 -> Mux/1, [engine_speed]  "Engine speed (rpm)"
  PS-Simulink Converter1/1 -> Product/1, Product1/1
  rad/s to rpm/1 -> Product/2
  Mux/1 -> [ICE_Meas]
  connections:
  Ideal Torque Sensor/LConn1 -- Engine/RConn1 -- Ideal Rotational Motion Sensor/LConn1
  Trans/RConn1 -- Ideal Torque Sensor/RConn1
  PS-Simulink Converter/LConn1 -- Ideal Torque Sensor/RConn2
  Ideal Rotational Motion Sensor/RConn2 -- PS-Simulink Converter1/LConn1
  Mechanical Rotational Reference/LConn1 -- Ideal Rotational Motion Sensor/RConn1

== system HEV_Model_PCT/Kph Demand/10-15 mode  ==
  Demux : Demux  Tag=STV Demux  Outputs=1
  FromWs : FromWorkspace  Tag=STV FromWs  VariableName=tuvar  SampleTime=0
      SigBuilderData=|
      | common.afterFinalStr = 'Extrapolate'
      | common.sampleTime = '0'
      | dataSet.timeRange = [0 660]
      | dataSet.name = '10-15 Mode Cycle'
      | sbobj.Groups.Name = '10-15 Mode Cycle'
      | sbobj.Groups.Signals.Name = 'Target speed'
      | sbobj.Groups.Signals.XData = [0 44 51 66 73 89 103 118 128 130 142 152 159 179 186 201 208 224 238 253 263 265 277 287 294 314 321 336 343 359 373 388 398 400 412 422 429 494 512 524 528 532 548 558 569 579 589 593 615 620 640 650 660]
      | sbobj.Groups.Signals.YData = [0 0 20 20 0 0 40 40 20 20 40 20 0 0 20 20 0 0 40 40 20 20 40 20 0 0 20 20 0 0 40 40 20 20 40 20 0 0 50 50 40 40 60 60 70 70 50 50 70 70 30 0 0]
  Target speed : Outport  Tag=STV Outport
  wires:
  Demux/1 -> Target speed/1
  FromWs/1 -> Demux/1

== system HEV_Model_PCT/Kph Demand/Vehicle Speed Controller ==
  Ref Spd : Inport
  Veh Spd : Inport  Port=2
  20Hz Lowpass Filter : TransferFcn  Denominator=[1/(2*pi*20) 1]
  Accel Ctrl : Scope  NumInputPorts=4
      settings: YMin=0~-0.05~-0.4~-5  YMax=0.08~0.1~0.4~5  SaveName=ScopeData11  MaxDataPoints=100  Decimation=decimation
  Ki : Gain  Gain=HEV_Param.Control.Veh_Spd.Ki
  Kp : Gain  Gain=HEV_Param.Control.Veh_Spd.Kp
  Limit : Saturate  UpperLimit=1  LowerLimit=0
  Limits [-5,5] : Integrator  LimitOutput=on  UpperSaturationLimit=5  LowerSaturationLimit=-5
  Mux : Mux  Inputs=2
  Sum : Sum  Inputs=-+|
  Sum1 : Sum  Inputs=++|
  Acc : Outport
  wires:
  Limit/1 -> Acc/1, Accel Ctrl/1
  Ref Spd/1 -> Sum/2, Mux/1
  Veh Spd/1 -> 20Hz Lowpass Filter/1, Mux/2
  Sum1/1 -> Limit/1, Accel Ctrl/2
  Sum/1 -> Ki/1, Kp/1, Accel Ctrl/3
  Ki/1 -> Limits [-5,5]/1
  Kp/1 -> Sum1/2
  Limits [-5,5]/1 -> Sum1/1
  20Hz Lowpass Filter/1 -> Sum/1
  Mux/1 -> Accel Ctrl/4

== system HEV_Model_PCT/Power Split Device /Sensor1 ==
  Ideal Rotational Motion Sensor : fl_lib/Mechanical/Mechanical Sensors/Ideal Rotational Motion Sensor  offset=0 rad
  Ideal Torque Sensor : fl_lib/Mechanical/Mechanical Sensors/Ideal Torque Sensor
  Mechanical Rotational Reference : fl_lib/Mechanical/Rotational Elements/Mechanical Rotational Reference
  PS-Simulink Converter : nesl_utility/PS-Simulink Converter  PhysicalDomain=network_engine_domain  SubClassName=ps_output  LeftPortType=input  RightPortType=output  PseudoPeriodic=off  Frequencies=[]  Unit=N*m  AffineConversion=off
  PS-Simulink Converter1 : nesl_utility/PS-Simulink Converter  PhysicalDomain=network_engine_domain  SubClassName=ps_output  LeftPortType=input  RightPortType=output  PseudoPeriodic=off  Frequencies=[]  Unit=rad/s  AffineConversion=off
  PG : PMIOPort  Port=1  Side=Right
  Sh : PMIOPort  Port=2  Side=Left
  tag scope: Carrier_Spd_radps=global, Carrier_Trq_Nm=global
  wires:
  PS-Simulink Converter/1 -> [Carrier_Trq_Nm]  "Carrier torque (Nm)"
  PS-Simulink Converter1/1 -> [Carrier_Spd_radps]
  connections:
  PG/RConn1 -- Ideal Torque Sensor/RConn1 -- Ideal Rotational Motion Sensor/RConn1
  Mechanical Rotational Reference/LConn1 -- Ideal Rotational Motion Sensor/LConn1
  PS-Simulink Converter/LConn1 -- Ideal Torque Sensor/RConn2
  PS-Simulink Converter1/LConn1 -- Ideal Rotational Motion Sensor/RConn2
  Sh/RConn1 -- Ideal Torque Sensor/LConn1

== system HEV_Model_PCT/Power Split Device /Sensor2 ==
  Ideal Rotational Motion Sensor : fl_lib/Mechanical/Mechanical Sensors/Ideal Rotational Motion Sensor  offset=0 rad
  Ideal Torque Sensor : fl_lib/Mechanical/Mechanical Sensors/Ideal Torque Sensor
  Mechanical Rotational Reference : fl_lib/Mechanical/Rotational Elements/Mechanical Rotational Reference
  PS-Simulink Converter : nesl_utility/PS-Simulink Converter  PhysicalDomain=network_engine_domain  SubClassName=ps_output  LeftPortType=input  RightPortType=output  PseudoPeriodic=off  Frequencies=[]  Unit=N*m  AffineConversion=off
  PS-Simulink Converter1 : nesl_utility/PS-Simulink Converter  PhysicalDomain=network_engine_domain  SubClassName=ps_output  LeftPortType=input  RightPortType=output  PseudoPeriodic=off  Frequencies=[]  Unit=rad/s  AffineConversion=off
  PG : PMIOPort  Port=1  Side=Right
  Sh : PMIOPort  Port=2  Side=Left
  tag scope: Ring_Spd_radps=global, Ring_Trq_Nm=global
  wires:
  PS-Simulink Converter/1 -> [Ring_Trq_Nm]  "Ring  torque (Nm)"
  PS-Simulink Converter1/1 -> [Ring_Spd_radps]  "Ring speed (rad/s)"
  connections:
  Ideal Rotational Motion Sensor/RConn1 -- PG/RConn1 -- Ideal Torque Sensor/RConn1
  Sh/RConn1 -- Ideal Torque Sensor/LConn1
  PS-Simulink Converter/LConn1 -- Ideal Torque Sensor/RConn2
  Mechanical Rotational Reference/LConn1 -- Ideal Rotational Motion Sensor/LConn1
  PS-Simulink Converter1/LConn1 -- Ideal Rotational Motion Sensor/RConn2

== system HEV_Model_PCT/Power Split Device /Sensor3 ==
  Ideal Rotational Motion Sensor : fl_lib/Mechanical/Mechanical Sensors/Ideal Rotational Motion Sensor  offset=0 rad
  Ideal Torque Sensor : fl_lib/Mechanical/Mechanical Sensors/Ideal Torque Sensor
  Mechanical Rotational Reference : fl_lib/Mechanical/Rotational Elements/Mechanical Rotational Reference
  PS-Simulink Converter : nesl_utility/PS-Simulink Converter  PhysicalDomain=network_engine_domain  SubClassName=ps_output  LeftPortType=input  RightPortType=output  PseudoPeriodic=off  Frequencies=[]  Unit=N*m  AffineConversion=off
  PS-Simulink Converter1 : nesl_utility/PS-Simulink Converter  PhysicalDomain=network_engine_domain  SubClassName=ps_output  LeftPortType=input  RightPortType=output  PseudoPeriodic=off  Frequencies=[]  Unit=rad/s  AffineConversion=off
  PG : PMIOPort  Port=1  Side=Right
  Sh : PMIOPort  Port=2  Side=Left
  tag scope: Sun_Spd_radps=global, Sun_Trq_Nm=global
  wires:
  PS-Simulink Converter1/1 -> [Sun_Spd_radps]
  PS-Simulink Converter/1 -> [Sun_Trq_Nm]  "Sun_Trq_Nm"
  connections:
  Sh/RConn1 -- Ideal Torque Sensor/LConn1
  PS-Simulink Converter1/LConn1 -- Ideal Rotational Motion Sensor/RConn2
  PS-Simulink Converter/LConn1 -- Ideal Torque Sensor/RConn2
  Mechanical Rotational Reference/LConn1 -- Ideal Rotational Motion Sensor/LConn1
  PG/RConn1 -- Ideal Torque Sensor/RConn1 -- Ideal Rotational Motion Sensor/RConn1

== system HEV_Model_PCT/Scopes/Batt DCDC Scopes ==
  Current : Scope  NumInputPorts=2
      settings: YMin=-0.5~-0.2  YMax=0~0  SaveName=ScopeData6  MaxDataPoints=100  Decimation=decimation*10
  Voltage : Scope  NumInputPorts=2
      settings: TimeRange=25  YMin=194~0  YMax=206~600  SaveName=ScopeData8  MaxDataPoints=100  Decimation=decimation
  DCDC Temp : Outport
  Batt Cell Temp : Outport  Port=2
  wires:
  [V_out] -> Voltage/2  "V_out"
  [I_in] -> Current/1  "I_in"
  [I_out] -> Current/2  "I_out"
  [V_in] -> Voltage/1
  [DCDC_SYS] -> DCDC Temp/1
  [Batt_Cell_Temp] -> Batt Cell Temp/1

== system HEV_Model_PCT/Scopes/Car Scopes ==
  Car : Scope  NumInputPorts=4
      settings: TimeRange=200  YMin=0~-20~-1~-40000  YMax=0.4~60~1~40000  SaveName=Car  Decimation=decimation
  wires:
  [Power] -> Car/3  "Power (Mot., Gen., Batt.)"
  [Torque] -> Car/2  "Drive torque (Ref., Meas.)"
  [VehSpd_kph] -> Car/4
  [Accelerator] -> Car/1  "Accelerator"

== system HEV_Model_PCT/Scopes/Drivetrain Scopes ==
  Mux6 : Mux  Inputs=2
  Speed (rad/s) : Scope  NumInputPorts=3
      settings: YMin=-100~-20~-200  YMax=500~120~1200  SaveName=ScopeData2  MaxDataPoints=100  Decimation=decimation
  Torque (Nm) : Scope  NumInputPorts=3
      settings: YMin=-50~-20~-10  YMax=150~100~40  SaveName=ScopeData4  MaxDataPoints=100  Decimation=decimation
  Vehicle Data : Scope
      settings: YMin=0  YMax=1  SaveName=Control_Logic1  MaxDataPoints=100  Decimation=decimation
  wires:
  [Ring_Spd_radps] -> Speed (rad/s)/2  "Ring speed (rad/s) - motor"
  [Sun_Spd_radps] -> Speed (rad/s)/3  "Sun speed (rad/s) - generator"
  [Ring_Trq_Nm] -> Torque (Nm)/2  "Ring torque (Nm) - motor"
  [Carrier_Spd_radps] -> Speed (rad/s)/1  "Carrier speed (rad/s) - engine (ICE)"
  [Sun_Trq_Nm] -> Torque (Nm)/3  "Sun torque (Nm) - generator"
  [Carrier_Trq_Nm] -> Torque (Nm)/1  "Carrier torque (Nm) - engine (ICE)"
  [FA_RPM] -> Mux6/1
  [RA_RPM] -> Mux6/2
  Mux6/1 -> Vehicle Data/1

== system HEV_Model_PCT/Scopes/Electricals Scopes ==
  Electricals : Scope  NumInputPorts=4
      settings: YMin=499~200~-150~99  YMax=501~500~100~100  SaveName=Electricals  Decimation=decimation
  Selector6 : Selector  InputPortWidth=8  Indices=[1 2]
  Selector7 : Selector  InputPortWidth=8  Indices=[3 4]
  Selector8 : Selector  InputPortWidth=8  Indices=[5 6 7]
  Selector9 : Selector  InputPortWidth=8  Indices=[8]
  V : Outport
  tag scope: SOC_out=global
  wires:
  Selector6/1 -> Electricals/1  "DC/DC converter Voltage (Reference, Measured)"
  Selector7/1 -> Electricals/2, V/1  "Voltage (DC bus, Battery)"
  Selector8/1 -> Electricals/3  "Current (Motor, Battery, Generator)"
  Selector9/1 -> Electricals/4, [SOC_out]
  [Electricals] -> Selector8/1, Selector9/1, Selector7/1, Selector6/1

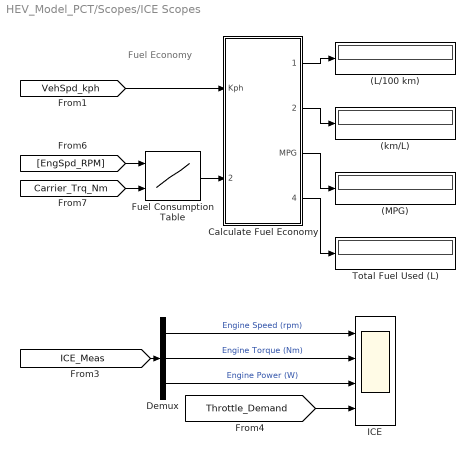
== system HEV_Model_PCT/Scopes/ICE Scopes ==
  note: Fuel Economy
  (L/100 km) : Display
      settings: Decimation=decimation
  (MPG) : Display
      settings: Decimation=decimation
  (km/L) : Display
      settings: Decimation=decimation
  Calculate Fuel Economy : Subsystem
  Demux : Demux  Outputs=3
  Fuel Consumption Table : Lookup2D  RowIndex=HEV_Param.ICE.FC.Speed_Vector  ColumnIndex=HEV_Param.ICE.FC.Torque_Vector  Table=HEV_Param.ICE.FC.Consumption_Table
  ICE : Scope  NumInputPorts=4
      settings: YMin=-500~-50~-5000~0  YMax=1500~250~20000~1  SaveName=ScopeData3  MaxDataPoints=100  Decimation=decimation
  Total Fuel Used (L) : Display
      settings: Decimation=decimation
  wires:
  [ICE_Meas] -> Demux/1
  Demux/1 -> ICE/1  "Engine Speed (rpm)"
  Demux/2 -> ICE/2  "Engine Torque (Nm)"
  Demux/3 -> ICE/3  "Engine Power (W)"
  [Throttle_Demand] -> ICE/4
  Calculate Fuel Economy/1(Liter/100Km) -> (L/100 km)/1
  Calculate Fuel Economy/3(MPG) -> (MPG)/1
  [VehSpd_kph] -> Calculate Fuel Economy/1(Kph)
  Calculate Fuel Economy/4(Fuel Used (L)) -> Total Fuel Used (L)/1
  Calculate Fuel Economy/2(Km/Liter) -> (km/L)/1
  Fuel Consumption Table/1 -> Calculate Fuel Economy/2(Fuel Flow g/s)
  [EngSpd_RPM] -> Fuel Consumption Table/1
  [Carrier_Trq_Nm] -> Fuel Consumption Table/2

== system HEV_Model_PCT/Scopes/Mode Logic ==
  Check State Logic : Scope  NumInputPorts=3
      settings: YMin=0~0~0  YMax=1~1~1  SaveName=Control_Logic  Decimation=decimation
  Mux5 : Mux  Inputs=2
  wires:
  [ICE_Enable] -> Mux5/1
  [engine_running] -> Mux5/2
  Mux5/1 -> Check State Logic/1
  [Mot_Enable] -> Check State Logic/2
  [Gen_Enable] -> Check State Logic/3

== system HEV_Model_PCT/Scopes/Motor Generator Scopes ==
  Control Scopes : Subsystem
  PMSM Generator Drive : Scope  NumInputPorts=3
      settings: YMin=-1~-1000~-150  YMax=1~3000~50  SaveName=Generator  Decimation=decimation
  PMSM Motor Drive : Scope  NumInputPorts=3
      settings: YMin=-1~-200~-400  YMax=1~600~400  SaveName=Motor  Decimation=decimation
  Selector : Selector  InputPortWidth=4  Indices=[1]
  Selector1 : Selector  InputPortWidth=4  Indices=[2]
  Selector2 : Selector  InputPortWidth=4  Indices=[3 4]
  Selector3 : Selector  InputPortWidth=4  Indices=[1]
  Selector4 : Selector  InputPortWidth=4  Indices=[2]
  Selector5 : Selector  InputPortWidth=4  Indices=[3 4]
  M : Outport
  G : Outport  Port=2
  wires:
  Selector1/1 -> PMSM Motor Drive/2, Control Scopes/1(In1), M/1  "Rotor speed (rpm)"
  Selector2/1 -> PMSM Motor Drive/3  "Electromagnetic Torque (Nm) [measured, reference]"
  Selector/1 -> PMSM Motor Drive/1  "Stator current (A)"
  [MotorDrive] -> Selector/1, Selector1/1, Selector2/1
  Selector4/1 -> PMSM Generator Drive/2, Control Scopes/2(In2), G/1  "Rotor speed (rpm)"
  Selector5/1 -> PMSM Generator Drive/3  "Electromagnetic Torque (Nm) [measured, reference]"
  Selector3/1 -> PMSM Generator Drive/1  "Stator current (A)"
  [GeneratorDrive] -> Selector5/1, Selector4/1, Selector3/1

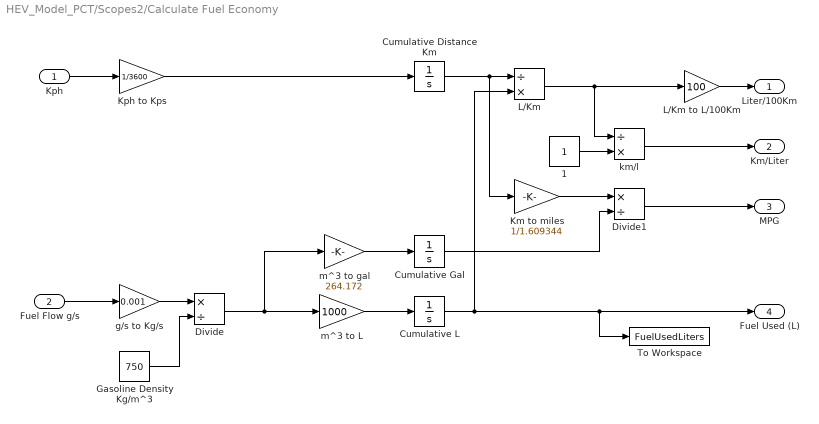
== system HEV_Model_PCT/Scopes2/Calculate Fuel Economy ==
  Kph : Inport
  Fuel Flow g/s : Inport  Port=2
  1 : Constant
  Cumulative Distance Km : Integrator  InitialCondition=eps
  Cumulative Gal : Integrator  InitialCondition=eps
  Cumulative L : Integrator  InitialCondition=eps
  Divide : Product  Inputs=*/
  Divide1 : Product  Inputs=*/
  Gasoline Density Kg/m^3 : Constant  Value=750
  Km to miles : Gain  Gain=1/1.609344
  Kph to Kps : Gain  Gain=1/3600
  L/Km : Product  Inputs=/*
  L/Km to L/100Km : Gain  Gain=100
  To Workspace : ToWorkspace  VariableName=FuelUsedLiters  SampleTime=-1
      settings: MaxDataPoints=1
  g/s to Kg/s : Gain  Gain=0.001
  km/l : Product  Inputs=/*
  m^3 to L : Gain  Gain=1000
  m^3 to gal : Gain  Gain=264.172
  Liter/100Km : Outport
  Km/Liter : Outport  Port=2
  MPG : Outport  Port=3
  Fuel Used (L) : Outport  Port=4
  wires:
  km/l/1 -> Km/Liter/1
  1/1 -> km/l/2
  Divide1/1 -> MPG/1
  L/Km to L/100Km/1 -> Liter/100Km/1
  Fuel Flow g/s/1 -> g/s to Kg/s/1
  Kph/1 -> Kph to Kps/1
  Cumulative Gal/1 -> Divide1/2
  Km to miles/1 -> Divide1/1
  L/Km/1 -> km/l/1, L/Km to L/100Km/1
  Cumulative Distance Km/1 -> Km to miles/1, L/Km/1
  Cumulative L/1 -> L/Km/2, Fuel Used (L)/1, To Workspace/1
  Kph to Kps/1 -> Cumulative Distance Km/1
  m^3 to gal/1 -> Cumulative Gal/1
  m^3 to L/1 -> Cumulative L/1
  Divide/1 -> m^3 to gal/1, m^3 to L/1
  Gasoline Density Kg/m^3/1 -> Divide/2
  g/s to Kg/s/1 -> Divide/1
